simulink model "StanfordArmModel"  (R2019b)
settings: Solver=FixedStepAuto  StartTime=0.0  StopTime=inf  RelTol=1e-3
libraries: simulink x8
settings Model: PacingRate=0.890000  Creator=crbon  LastModifiedBy=Chris

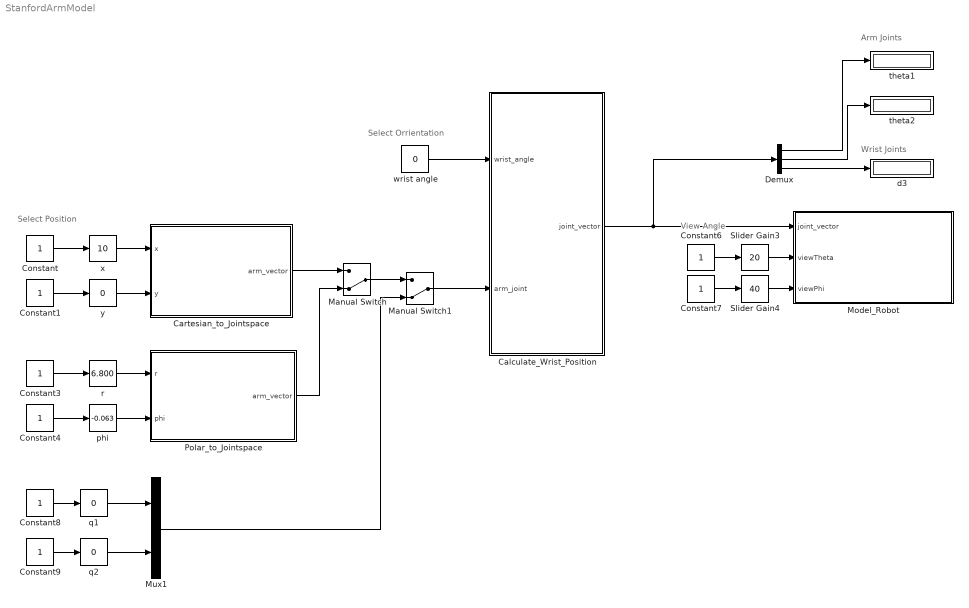
== system StanfordArmModel ==
  note: View Angle
  note: Select Orrientation
  note: Select Position
  note: Wrist Joints
  note: Arm Joints
  Calculate_Wrist_Position : MATLAB Function  TreatAsAtomicUnit=on
  Cartesian_to_Jointspace : MATLAB Function  TreatAsAtomicUnit=on
  Constant{,1,3..4,6..9} (8 alike) : Constant
  Demux : Demux  Outputs=3
  Manual Switch : ManualSwitch  CurrentSetting=0
  Manual Switch1 : ManualSwitch  CurrentSetting=0
  Model_Robot : MATLAB Function  TreatAsAtomicUnit=on
  Mux1 : Mux  Inputs=2
  Polar_to_Jointspace : MATLAB Function  TreatAsAtomicUnit=on
  Slider Gain3 : simulink/Math Operations/Slider Gain  gain=20  low=-90  high=90
  Slider Gain4 : simulink/Math Operations/Slider Gain  gain=40  low=-90  high=90
  d3 : Display
  phi : simulink/Math Operations/Slider Gain  gain=-0.063  low=-3.15  high=3.15
  q1 : simulink/Math Operations/Slider Gain  gain=0  low=-3.14  high=3.14
  q2 : simulink/Math Operations/Slider Gain  gain=0  low=-3.14  high=3.14
  "r " : simulink/Math Operations/Slider Gain  gain=6.800  low=2  high=10
  theta1 : Display
  theta2 : Display
  wrist angle : Constant  Value=0
  x : simulink/Math Operations/Slider Gain  gain=10  low=-12  high=12
  y : simulink/Math Operations/Slider Gain  gain=0  low=-12  high=12
  wires:
  Slider Gain4/1 -> Model_Robot/3(viewPhi)
  Slider Gain3/1 -> Model_Robot/2(viewTheta)
  Constant7/1 -> Slider Gain4/1
  Constant6/1 -> Slider Gain3/1
  Constant4/1 -> phi/1
  phi/1 -> Polar_to_Jointspace/2(phi)
  wrist angle/1 -> Calculate_Wrist_Position/1(wrist_angle)
  y/1 -> Cartesian_to_Jointspace/2(y)
  Polar_to_Jointspace/1(arm_vector) -> Manual Switch/2
  Constant/1 -> x/1
  Cartesian_to_Jointspace/1(arm_vector) -> Manual Switch/1
  "r "/1 -> Polar_to_Jointspace/1(r)
  x/1 -> Cartesian_to_Jointspace/1(x)
  Constant3/1 -> "r "/1
  Constant1/1 -> y/1
  Manual Switch/1 -> Manual Switch1/1
  Calculate_Wrist_Position/1(joint_vector) -> Demux/1, Model_Robot/1(joint_vector)
  Demux/1 -> theta1/1
  Demux/3 -> d3/1
  Demux/2 -> theta2/1
  q2/1 -> Mux1/2
  Constant9/1 -> q2/1
  q1/1 -> Mux1/1
  Mux1/1 -> Manual Switch1/2
  Constant8/1 -> q1/1
  Manual Switch1/1 -> Calculate_Wrist_Position/2(arm_joint)

== matlab function StanfordArmModel/Cartesian_to_Jointspace ==
  data: x input; y input; arm_vector output
% creates a joint vector for the position of the stanford arm from 
% a cartesian input; doesn't calculate wrist angles or EOAT
function arm_vector  = Cartesian_to_Jointspace(x,y)
%% initialize
arm_vector = zeros(1,2);
L1=4;
L2=6;

%% theta2
theta2 = acos((x^2+y^2-L1^2-L2^2)/(2*L1*L2));
arm_vector(2) = theta2;

%% theta1
theta1 = atan2(y,x) - atan2(L2*sin(theta2),L1+L2*cos(theta2));
arm_vector(1) = theta1;

== matlab function StanfordArmModel/Model_Robot ==
  data: joint_vector input; viewTheta input; viewPhi input
function Model_Robot(joint_vector, viewTheta, viewPhi)

%% Unpack Joint Vector
theta = joint_vector;
L1 = 8;
L2 = 6;
EOA = 4;
L = [0 L1 L2 EOA];

%% Define Links/ Robot Shapes
origin = [0;0;0];

Base  = [...
         -1  -1  -1  -1  -1   1   1  -1   1   1  -1   1   1  -1   1   1;...
          1  -1  -1   1   1   1   1   1   1  -1  -1  -1  -1  -1  -1   1;...
        -15 -15  -1  -1 -15 -15  -1  -1  -1  -1  -1  -1 -15 -15 -15 -15;...
];

Link1 = [...
          1  -1  -1   1   1   1   1   1   1  -1  -1  -1  -1  -1  -1   1;...
          1   1  -1  -1   1   1  -1  -1  -1  -1  -1  -1   1   1   1   1;...
         -1  -1  -1  -1  -1   1   1  -1   1   1  -1   1   1  -1   1   1;...
];

L1rod = [...
          1  L1  L1   1   1   1   1   1   1  L1  L1  L1  L1  L1  L1   1;...
         .5  .5 -.5 -.5  .5  .5 -.5 -.5 -.5 -.5 -.5 -.5  .5  .5  .5  .5;...
        -.5 -.5 -.5 -.5 -.5  .5  .5 -.5  .5  .5 -.5  .5  .5 -.5  .5  .5;...
];

Link2 = [...
          1  -1  -1   1   1   1   1   1   1  -1  -1  -1  -1  -1  -1   1;...
          1   1  -1  -1   1   1  -1  -1  -1  -1  -1  -1   1   1   1   1;...
         -1  -1  -1  -1  -1   1   1  -1   1   1  -1   1   1  -1   1   1;...
];

L2rod = [...
          1  L2  L2   1   1   1   1   1   1  L2  L2  L2  L2  L2  L2   1;...
         .5  .5 -.5 -.5  .5  .5 -.5 -.5 -.5 -.5 -.5 -.5  .5  .5  .5  .5;...
        -.5 -.5 -.5 -.5 -.5  .5  .5 -.5  .5  .5 -.5  .5  .5 -.5  .5  .5;...
];

Link3 = [...
          1  -1  -1   1   1   1   1   1   1  -1  -1  -1  -1  -1  -1   1;...
          1   1  -1  -1   1   1  -1  -1  -1  -1  -1  -1   1   1   1   1;...
         -1  -1  -1  -1  -1   1   1  -1   1   1  -1   1   1  -1   1   1;...
];

L3rod = [...
          1  EOA EOA  1   1   1   1   1   1  EOA EOA EOA EOA EOA EOA  1;...
         .5  .5 -.5 -.5  .5  .5 -.5 -.5 -.5 -.5 -.5 -.5  .5  .5  .5  .5;...
        -.5 -.5 -.5 -.5 -.5  .5  .5 -.5  .5  .5 -.5  .5  .5 -.5  .5  .5;...
];

% shape of axis figure for base and EOAT
axes  = 2*[...
         0 1.5 0  0  0  0  0;...
         0  0  0 1.5 0  0  0;...
         0  0  0  0  0 1.5 0;...
];

%% Transform Link 1
BaseLink1= TRANSRRR(Link1 ,theta(1), L(1));
Link1rod = TRANSRRR(L1rod ,theta(1), L(1));
BaseLink1O = TRANSRRR(axes,theta(1),L(1));


%% Transform Link 2
Link12   = TRANSRRR(Link2 ,theta(2), L(2));
BaseLink2= TRANSRRR(Link12,theta(1), L(1));

L2rod    = TRANSRRR(L2rod ,theta(2), L(2));
Link2rod = TRANSRRR(L2rod ,theta(1), L(1));
BaseLink2O = TRANSRRR(TRANSRRR(axes,theta(2),L(2)),theta(1),L(1));

%% Transform Link 3
Link23   = TRANSRRR(Link3 ,theta(3), L(3));
Link13   = TRANSRRR(Link23,theta(2), L(2));
BaseLink3= TRANSRRR(Link13,theta(1), L(1));

L3rod    = TRANSRRR(L3rod ,theta(3), L(3));
L3rod    = TRANSRRR(L3rod ,theta(2), L(2));
Link3rod = TRANSRRR(L3rod ,theta(1), L(1));
BaseLink3O = TRANSRRR(TRANSRRR(TRANSRRR(axes,theta(3),L(3)),theta(2),L(2)),theta(1),L(1));




%% Plotting
plot3(Base(1,:),Base(2,:),Base(3,:),'k-')
axis([-5 20 -5 10 -5 10]);
grid on
hold on
plot3(BaseLink1(1,:),BaseLink1(2,:),BaseLink1(3,:),'b-', 'LineWidth', 2)
plot3(Link1rod(1,:), Link1rod(2,:), Link1rod(3,:), 'b-', 'LineWidth', 2)
plot3(BaseLink2(1,:),BaseLink2(2,:),BaseLink2(3,:),'g-', 'LineWidth', 2)
plot3(Link2rod(1,:), Link2rod(2,:), Link2rod(3,:), 'g-', 'LineWidth', 2)
plot3(BaseLink3(1,:),BaseLink3(2,:),BaseLink3(3,:),'k-', 'LineWidth', 2)
plot3(Link3rod(1,:), Link3rod(2,:), Link3rod(3,:), 'k-', 'LineWidth', 2)
plot3(BaseLink1O(1,:), BaseLink1O(2,:), BaseLink1O(3,:), 'r-', 'LineWidth', 4)
plot3(BaseLink2O(1,:), BaseLink2O(2,:), BaseLink2O(3,:), 'r-', 'LineWidth', 4)
plot3(BaseLink3O(1,:), BaseLink3O(2,:), BaseLink3O(3,:), 'r-', 'LineWidth', 4)

xlabel('X');
ylabel('Y');
zlabel('Z');
view(viewTheta,viewPhi);
set(gcf,'color','w');
hold off

end

== matlab function StanfordArmModel/Polar_to_Jointspace ==
  data: r input; phi input; arm_vector output
% creates a joint vector for the position of the stanford arm from 
% a spherical input; doesn't calculate wrist angles or EOAT
function arm_vector  = Spherical_to_Jointspace(r,phi)
%% initialize
arm_vector = zeros(1,2);
L1=4;
L2=6;

%% calculate cartesian
x = r*cos(phi);
y = r*sin(phi);

%% theta2
theta2 = acos((r^2-L1^2-L2^2)/(2*L1*L2));
arm_vector(2) = theta2;

%% theta1
theta1 = phi - atan2(L2*sin(theta2),L1+L2*cos(theta2));
arm_vector(1) = theta1;

== matlab function StanfordArmModel/Calculate_Wrist_Position ==
  data: wrist_angle input; arm_joint input; joint_vector output
function joint_vector  = Calculate_Wrist_Position(wrist_angle, arm_joint)

%%Initialize Joint Vector
joint_vector = zeros(1,3);

%% Unpack Joint Vector
theta1 = arm_joint(1);
theta2 = arm_joint(2);

%% Calculate Wrist Joint
theta3 = wrist_angle-theta1-theta2;
    
%% Make Joint Vector
joint_vector(1:3) = [theta1;theta2;theta3];

end
